simulink model "Model_9_linear"  (R2018a)
settings: Solver=VariableStepAuto  StartTime=0.0  StopTime=10.0  RelTol=1e-3
values from neighbouring files (symbols this model uses):
  deadzone_u = 2e-1    (= 0.2)    [CEE_10.m]    (also in CEE_10_performance.m; CEE_10_unc.m; CEE_11.m; CEE_9.m = 0.1)
  L = lqe(A, G, C, Qe, Re)    [CEE_10.m]    (also in CEE_10_performance.m; CEE_10_unc.m; CEE_11.m; CEE_9.m)
  pulse = 4    [CEE_10.m]    (also in CEE_10_performance.m; CEE_10_unc.m; CEE_9.m; CEE_9_performance.m)
  saturation_u = 5    [CEE_10.m]    (also in CEE_10_performance.m; CEE_10_unc.m; CEE_11.m; CEE_9.m)
  x0 = [50,0,10,0,0]'*pi/180    [CEE_10.m]    (also in CEE_10_performance.m; CEE_11.m; CEE_9.m; CEE_9_performance.m)
undefined symbols (not defined in the file or in its folder): A, B, C, K
settings Model: Creator=miguelsilva  LastModifiedBy=leonardopedroso
settings DebuggingCC: LibraryContextMissingDiagnostic=warning
settings SFSimCC: SimUseLocalCustomCode=on
settings RTWCC: RTWUseLocalCustomCode=on

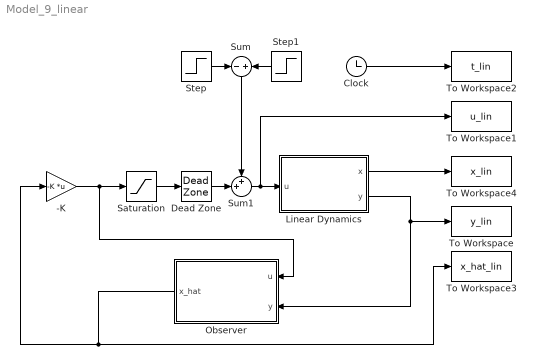
== system Model_9_linear ==
  -K : Gain  Gain=-K  Multiplication=Matrix(K*u) (u vector)
  Clock : Clock
  "Dead Zone " : DeadZone  LowerValue=-deadzone_u  UpperValue=deadzone_u  SaturateOnIntegerOverflow=on
  Linear Dynamics : Subsystem
  "Observer " : Subsystem
  "Saturation " : Saturate  UpperLimit=saturation_u  LowerLimit=-saturation_u
  Step : Step  Time=5.1  After=pulse  SampleTime=0
  Step1 : Step  Time=5  After=pulse  SampleTime=0
  Sum : Sum  Inputs=-|+
  Sum1 : Sum  Inputs=++|
  To Workspace : ToWorkspace  VariableName=y_lin  SampleTime=-1
  To Workspace1 : ToWorkspace  VariableName=u_lin  SampleTime=-1
  To Workspace2 : ToWorkspace  VariableName=t_lin  SampleTime=-1
  To Workspace3 : ToWorkspace  VariableName=x_hat_lin  SampleTime=-1
  To Workspace4 : ToWorkspace  VariableName=x_lin  SampleTime=-1
  wires:
  Clock/1 -> To Workspace2/1
  Linear Dynamics/1(x) -> To Workspace4/1
  Linear Dynamics/2(y) -> To Workspace/1, "Observer "/2("y ")
  "Observer "/1(x_hat) -> -K/1, To Workspace3/1
  -K/1 -> "Observer "/1(u), "Saturation "/1
  "Saturation "/1 -> "Dead Zone "/1
  Step/1 -> Sum/1
  Step1/1 -> Sum/2
  Sum/1 -> Sum1/1
  "Dead Zone "/1 -> Sum1/2
  Sum1/1 -> To Workspace1/1, Linear Dynamics/1(u)

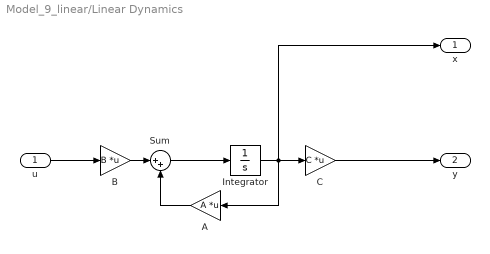
== system Model_9_linear/Linear Dynamics ==
  u : Inport
  A : Gain  Gain=A  Multiplication=Matrix(K*u) (u vector)
  B : Gain  Gain=B  Multiplication=Matrix(K*u) (u vector)
  C : Gain  Gain=C  Multiplication=Matrix(K*u) (u vector)
  Integrator : Integrator  InitialCondition=x0
  Sum : Sum  Inputs=|++
  x : Outport
  y : Outport  Port=2
  wires:
  u/1 -> B/1
  C/1 -> y/1
  B/1 -> Sum/1
  Sum/1 -> Integrator/1
  A/1 -> Sum/2
  Integrator/1 -> x/1, C/1, A/1

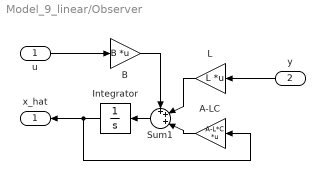
== system Model_9_linear/Observer  ==
  u : Inport
  "y " : Inport  Port=2
  A-LC : Gain  Gain=A-L*C  Multiplication=Matrix(K*u) (u vector)
  B : Gain  Gain=B  Multiplication=Matrix(K*u) (u vector)
  Integrator : Integrator  InitialCondition=zeros(5,1)
  L : Gain  Gain=L  Multiplication=Matrix(K*u) (u vector)
  Sum1 : Sum  Inputs=+++|
  x_hat : Outport
  wires:
  Integrator/1 -> x_hat/1, A-LC/1
  L/1 -> Sum1/2
  "y "/1 -> L/1
  Sum1/1 -> Integrator/1
  A-LC/1 -> Sum1/3
  B/1 -> Sum1/1
  u/1 -> B/1
